simulink model "DCDC_4_5"  (R2012b)
settings: Solver=ode23  StartTime=0.0  StopTime=1370  FixedStep=0.1  MaxStep=0.005  RelTol=1e-6
undefined symbols (not defined in the file): Hydride, Metal, Nickel
libraries: powerlib x15, simulink x4, electricdrivelib x1
settings Model: Creator=Administrator  LastModifiedBy=Administrator
settings DataIOCC: SignalLoggingSaveFormat=ModelDataLogs
settings DebuggingCC: FcnCallInpInsideContextMsg=UseLocalSettings  StrictBusMsg=Warning
settings GRTTargetCC: CombineOutputUpdateFcns=off  GRTInterface=on

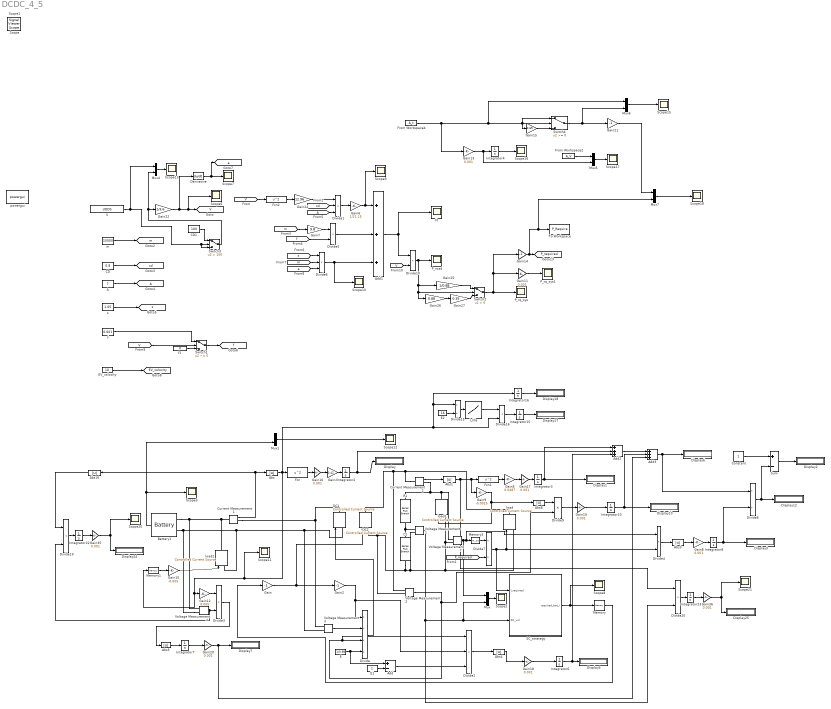
== system DCDC_4_5 ==
  A : Constant  Value=7
  Abs{,1,3..5,8,16} (7 alike) : Abs
  Add : Sum  Inputs=+-
  Add1 : Sum  Inputs=+++
  Add2 : Sum  Inputs=+++
  Add3 : Sum  Inputs=+++
  Battery1 : electricdrivelib/Extra Sources/Battery  BatType=Nickel-Metal-Hydride  ShowDetailedParameters=on  NomV=576  NomQ=160  SOC=90  PresetModel=off  MaxQ=17.2308  FullV=306.2712  Dis_rate=3.2  R=0.09  Normal_OP=15.3846  expZone="[282.0339           3.2]"  Dis_Char=off  current=[1.5 3]  Units=Ampere-hour  Batt_Tr=30
  C1 : powerlib/Elements/Series RLC Branch  LConnTagsString=__new0  RConnTagsString=__new0  BranchType=C  Resistance=1  Inductance=1e-3  SetiL0=off  InitialCurrent=0  Capacitance=14.1  Setx0=on  InitialVoltage=400  Measurements=Branch voltage
  CD : Constant  Value=0.8
  CD1 : Constant  Value=100
  Constant : Constant
  Current Measurement1 : powerlib/Measurements/Current Measurement  PhasorSimulation=off  OutputType=Complex  PSBequivalent=0
  Current Measurement2 : powerlib/Measurements/Current Measurement  PhasorSimulation=off  OutputType=Complex  PSBequivalent=0
  DC1 : powerlib/Electrical Sources/Controlled Current Source  Initialize=on  Source_Type=AC  Amplitude=0  Phase=0  Frequency=0  Measurements=None
  DC2 : powerlib/Electrical Sources/Controlled Current Source  Initialize=on  Source_Type=AC  Amplitude=0  Phase=0  Frequency=0  Measurements=None
  Derivative : Derivative
  Display{,1..4,6..7,10,12,17..18,24..25} (13 alike) : Display
  Divide : Product  Inputs=*/**
  Divide1 : Product  Inputs=***
  Divide{3..5,9..10,16,19..20} (8 alike) : Product  Inputs=**
  Divide15 : Product  Inputs=*/
  Divide2 : Product  Inputs=***
  Divide6 : Product  Inputs=***
  Divide7 : Product  Inputs=/*
  Divide8 : Product  Inputs=*/
  E : Constant  Value=1/0.98
  E1 : Constant
  E2 : Constant  Value=16
  EV_volocity : Constant  Value=10
  Fcn : Fcn  Expr=u^2
  Fcn1 : Fcn  Expr=u^2
  Fcn2 : Fcn  Expr=u^2
  From Workspace2 : FromWorkspace  VariableName=A_V  SampleTime=0
  From Workspace4 : FromWorkspace  VariableName=A_t  SampleTime=0
  Ft : Scope
      settings: SaveName=ScopeData9
  Gain{,2,14,21} (4 alike) : Gain  Gain=-1
  Gain10 : Gain  Gain=-0.005
  Gain{8,11,13,16..20,35..36} (10 alike) : Gain  Gain=0.001
  Gain12 : Gain  Gain=0.005
  Gain15 : Gain  Gain=0.65
  Gain22 : Gain  Gain=1/3.6
  Gain24 : Gain  Gain=12.96
  Gain25 : Gain  Gain=1/0.88
  Gain26 : Gain  Gain=0.88
  Gain27 : Gain  Gain=0.35
  Gain4 : Gain  Gain=0.42
  Gain5 : Gain  Gain=0.0487
  Gain6 : Gain  Gain=1/21.15
  Gain7 : Gain  Gain=9.8
  Gain9 : Gain  Gain=-0.0025
  I_life : Lookup  InputValues=[1,2,3,4,5]  Table=[1,1.0222,1.033,1.09,1.179]
  Integrator{2..4,6..8,10,15..16,22..23} (11 alike) : Integrator
  Memory : Memory
  Memory1 : Memory
  Memory3 : Memory  X0=380
  Mux{,1,4..7} (6 alike) : Mux  Inputs=2
  P_road : Scope
      settings: SaveName=P_road
  P_rq_sys : Scope
      settings: SaveName=ScopeData11
  P_rq_sys1 : Scope
      settings: SaveName=ScopeData10
  R1 : powerlib/Elements/Series RLC Branch  LConnTagsString=__new0  RConnTagsString=__new0  BranchType=R  Resistance=0.0487  Inductance=1e-3  SetiL0=off  InitialCurrent=0  Capacitance=1e-6  Setx0=off  InitialVoltage=0  Measurements=None
  SC_strategy : Subsystem
  Scope{2..3,6..13,15..18,20..21} (16 alike) : Scope
      Scope10 settings: SaveName=ScopeData12
      Scope11 settings: SaveName=ScopeData4
      Scope12 settings: TimeRange=206.5472513897466  YMin=-57.18262806236083  YMax=152.5055679287305
      Scope13 settings: SaveName=ScopeData8
      Scope15 settings: SaveName=ScopeData13
      Scope16 settings: SaveName=ScopeData14
      Scope17 settings: SaveName=ScopeData15
      Scope18 settings: SaveName=ScopeData16
      Scope2 settings: TimeRange=1600  YMin=240  YMax=420  SaveName=ScopeData2
      Scope20 settings: SaveName=ScopeData18
      Scope21 settings: SaveName=ScopeData19
      Scope3 settings: SaveName=ScopeData3
      Scope6 settings: SaveName=ScopeData17
      Scope7 settings: SaveName=ScopeData20
      Scope8 settings: SaveName=ScopeData5
      Scope9 settings: SaveName=ScopeData21
  Sum : Sum  Inputs=+-
  Switch1 : Switch  Criteria=u2 ~= 0
  Switch2 : Switch  Criteria=u2 > Threshold
  Switch3 : Switch  Criteria=u2 > Threshold  Threshold=100
  Switch4 : Switch
  To Workspace : ToWorkspace  VariableName=P_Require  SampleTime=-1
  V : FromWorkspace  VariableName=UDDS  SampleTime=0
  Voltage Measurement{1..4,7} (5 alike) : powerlib/Measurements/Voltage Measurement  PhasorSimulation=off  OutputType=Complex  PSBequivalent=0
  f : Constant  Value=0.001
  f1 : Constant  Value=0
  load : powerlib/Electrical Sources/Controlled Current Source  Initialize=on  Source_Type=AC  Amplitude=0  Phase=0  Frequency=0  Measurements=None
  load1 : powerlib/Electrical Sources/Controlled Current Source  Initialize=on  Source_Type=AC  Amplitude=0  Phase=0  Frequency=0  Measurements=None
  load2 : powerlib/Electrical Sources/Controlled Current Source  Initialize=on  Source_Type=AC  Amplitude=0  Phase=0  Frequency=0  Measurements=None
  m : Constant  Value=15000
  powergui : powerlib/powergui  Priority=1  SimulationMode=Discrete  SolverType=Tustin  SampleTime=0.01  frequency=60  SPID=off  DisableSnubberDevices=off  DisableRonSwitches=off  DisableVfSwitches=off  SwTol=0  Interpol=off  DisplayEquations=off  FunctionMessages=off  frequencyindice=0  Pbase=100e6  ErrMax=1e-4  Iterations=50  UnitsV=kV  UnitsW=MW  echomessages=off  HookPort=off  EnableUseOfTLC=off  x0status=blocks  RestoreLinks=warning  ResistiveCurrentMeasurement=off  Ylog=off  Xlog=on  ShowGrid=off  save=off  variable=ZData  ZoomFFT=off  StartTime=0.0  cycles=1  DisplayStyle=1  FreqAxis=off  MaxFrequency=1000  frequencyindicesteady=1  display=off  methode=off
  s : Constant  Value=1.05
  Scope : SignalViewerScope  IOType=viewer  RefreshTime=0.035000
  Scope1 : SignalViewerScope  IOType=viewer  RefreshTime=0.035000
  tag scope: A=global, EV_volocity=global, P_required=global, V=global, a=global, cd=global, f=global, m=global, s=global
  wires:
  Divide7/1 -> SC_strategy/1(I_requried), load/1, Divide4/2
  Battery1/1 -> Mux1/2, Scope3/1
  Voltage Measurement2/1 -> Divide/3, Divide2/1, Divide9/2
  Voltage Measurement1/1 -> Divide20/2, SC_strategy/2(SC_vol), Mux/2
  E/1 -> Divide/4, Add/1
  Voltage Measurement3/1 -> Divide/2
  Divide/1 -> DC1/1
  SC_strategy/1(required_bat_I) -> Memory/1, Scope8/1
  Memory/1 -> Gain/1
  Gain/1 -> DC2/1, Gain2/1
  Gain2/1 -> Divide/1, Divide2/2
  Current Measurement1/1 -> Abs/1, Abs16/1
  Current Measurement2/1 -> Abs1/1
  Abs/1 -> Fcn/1, Divide16/2, Divide15/1, Integrator16/1, Gain12/1, Memory1/1, Scope11/1
  Fcn/1 -> Gain16/1
  Gain4/1 -> Integrator2/1
  Integrator2/1 -> Display/1, Add2/2
  Fcn1/1 -> Gain5/1
  Gain5/1 -> Gain17/1
  Abs1/1 -> Fcn1/1, Gain9/1, Divide20/1
  Integrator3/1 -> Display1/1, Add2/1
  E1/1 -> Add/2
  Add/1 -> Divide2/3
  Abs4/1 -> Gain18/1
  Integrator6/1 -> Display4/1, Add2/3
  Divide2/1 -> Abs4/1
  Gain9/1 -> load1/1, Abs8/1
  Gain10/1 -> load2/1
  Voltage Measurement4/1 -> Divide3/2, Divide19/2
  Integrator7/1 -> Gain20/1
  Divide3/1 -> Abs5/1
  Abs5/1 -> Integrator7/1
  Gain12/1 -> Divide3/1
  [P_required] -> Divide7/2
  Voltage Measurement7/1 -> Divide4/1, Memory3/1, Mux/1
  Memory1/1 -> Gain10/1
  Memory3/1 -> Divide7/1
  Divide9/1 -> Gain19/1
  Integrator10/1 -> Display10/1, Add3/2
  Abs8/1 -> Divide9/1
  Divide4/1 -> Abs3/1
  Abs3/1 -> Gain8/1
  Integrator8/1 -> Display3/1, Divide8/2
  Gain8/1 -> Integrator8/1
  Gain16/1 -> Gain4/1
  Gain17/1 -> Integrator3/1
  Gain18/1 -> Integrator6/1
  Gain19/1 -> Integrator10/1
  Gain20/1 -> Display7/1, Add3/3
  Add2/1 -> Add3/1
  Add3/1 -> Divide8/1, Display6/1
  Divide8/1 -> Display12/1, Sum/2
  Mux1/1 -> Scope12/1
  Divide15/1 -> I_life/1
  E2/1 -> Divide15/2
  I_life/1 -> Divide16/1
  Divide16/1 -> Integrator15/1
  Integrator15/1 -> Display17/1
  Integrator16/1 -> Display18/1
  Divide19/1 -> Integrator22/1
  Integrator22/1 -> Gain35/1
  Gain35/1 -> Scope20/1, Display24/1
  Abs16/1 -> Divide19/1
  Divide20/1 -> Integrator23/1
  Integrator23/1 -> Gain36/1
  Gain36/1 -> Scope21/1, Display25/1
  Mux/1 -> Scope2/1
  V/1 -> Mux4/1, Switch3/3, Switch3/2
  m/1 -> [m]
  CD/1 -> [cd]
  A/1 -> [A]
  s/1 -> [s]
  Derivative/1 -> Scope7/1, [a]
  [V] -> Fcn2/1
  Fcn2/1 -> Gain24/1
  [cd] -> Divide1/2
  Divide1/1 -> Gain6/1
  Gain6/1 -> Add1/1, Scope9/1
  [m] -> Gain7/1
  Gain7/1 -> Divide5/1
  [f] -> Divide5/2
  [A] -> Divide1/3
  Divide5/1 -> Add1/2
  [s] -> Divide6/1
  [m] -> Divide6/2
  [a] -> Divide6/3
  Divide6/1 -> Add1/3, Scope10/1
  Add1/1 -> Ft/1, Divide10/1
  f/1 -> Switch1/1
  [V] -> Switch1/2
  f1/1 -> Switch1/3
  Switch1/1 -> [f]
  Gain22/1 -> Derivative/1, [V], Scope6/1
  [V] -> Divide10/2
  Gain24/1 -> Divide1/1
  Divide10/1 -> P_road/1, Gain25/1, Switch2/2, Gain26/1
  Gain25/1 -> Switch2/1
  Gain26/1 -> Gain27/1
  Switch2/1 -> P_rq_sys/1, Gain11/1, Gain14/1
  Gain27/1 -> Switch2/3
  EV_volocity/1 -> [EV_volocity]
  Gain14/1 -> Mux7/2, To Workspace/1, [P_required]
  Gain11/1 -> P_rq_sys1/1
  CD1/1 -> Switch3/1
  Switch3/1 -> Mux4/2, Gain22/1
  Mux4/1 -> Scope13/1
  Gain13/1 -> Integrator4/1, Mux5/2
  Integrator4/1 -> Scope16/1
  From Workspace4/1 -> Gain15/1, Switch4/1, Switch4/2, Mux6/1, Gain13/1
  From Workspace2/1 -> Mux5/1
  Mux5/1 -> Scope17/1
  Switch4/1 -> Gain21/1, Mux6/2
  Gain15/1 -> Switch4/3
  Mux6/1 -> Scope15/1
  Gain21/1 -> Mux7/1
  Mux7/1 -> Scope18/1
  Constant/1 -> Sum/1
  Sum/1 -> Display2/1
  connections:
  Current Measurement2/LConn1 -- load/RConn1 -- DC2/RConn1 -- Voltage Measurement2/LConn1
  C1/LConn1 -- Voltage Measurement1/LConn1 -- R1/RConn1
  load/LConn1 -- load1/LConn1 -- Voltage Measurement7/LConn2 -- DC2/LConn1 -- Voltage Measurement2/LConn2 -- C1/RConn1 -- Voltage Measurement1/LConn2
  Current Measurement1/RConn1 -- Voltage Measurement3/LConn1 -- DC1/RConn1
  Voltage Measurement4/LConn2 -- Battery1/LConn2 -- Voltage Measurement3/LConn2 -- DC1/LConn1 -- load2/LConn1
  Battery1/LConn1 -- Voltage Measurement4/LConn1 -- load2/RConn1 -- Current Measurement1/LConn1
  Voltage Measurement7/LConn1 -- load1/RConn1 -- Current Measurement2/RConn1 -- R1/LConn1

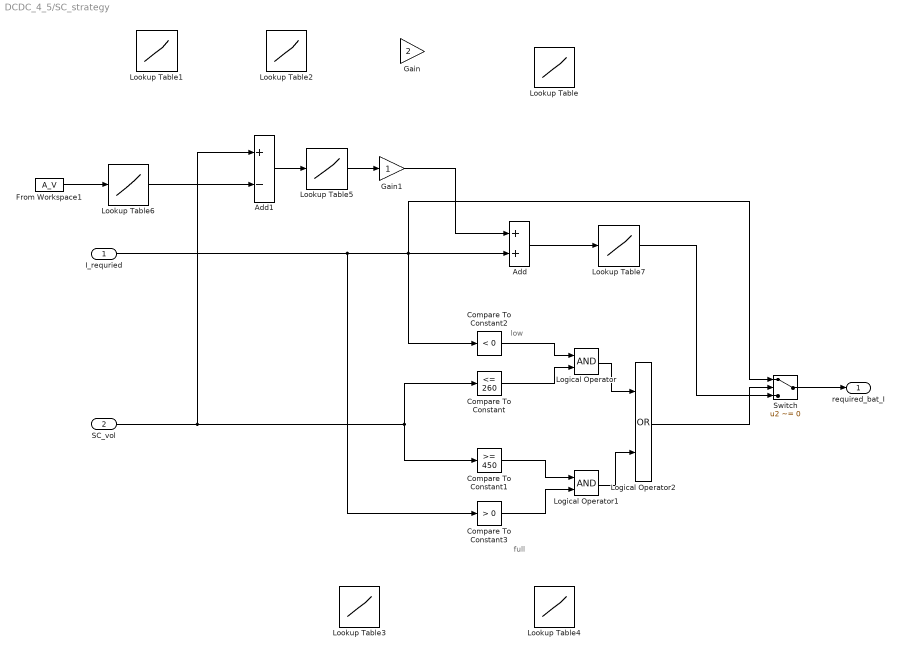
== system DCDC_4_5/SC_strategy ==
  note: full
  note: low
  I_requried : Inport
  SC_vol : Inport  Port=2
  Add : Sum
  Add1 : Sum  Inputs=+-
  Compare To Constant : simulink/Logic and Bit Operations/Compare To Constant  relop=<=  const=260  OutDataTypeStr=uint8  ZeroCross=off
  Compare To Constant1 : simulink/Logic and Bit Operations/Compare To Constant  relop=>=  const=450  OutDataTypeStr=uint8  ZeroCross=off
  Compare To Constant2 : simulink/Logic and Bit Operations/Compare To Constant  relop=<  const=0  OutDataTypeStr=uint8  ZeroCross=off
  Compare To Constant3 : simulink/Logic and Bit Operations/Compare To Constant  relop=>  const=0  OutDataTypeStr=uint8  ZeroCross=off
  From Workspace1 : FromWorkspace  VariableName=A_V  SampleTime=0
  Gain : Gain  Gain=2
  Gain1 : Gain
  Logical Operator : Logic  AllPortsSameDT=off  OutDataTypeStr=boolean
  Logical Operator1 : Logic  AllPortsSameDT=off  OutDataTypeStr=boolean
  Logical Operator2 : Logic  Operator=OR  AllPortsSameDT=off  OutDataTypeStr=boolean
  Lookup Table : Lookup  InputValues=[-260,-180,-100,-40,-20,-10,0,10,20,40,100,180,260]  Table=[-60,-30,-0,0,0,0,0,0,0,0,0,30,60]
  Lookup Table1 : Lookup  InputValues=[0,10,20,35,50,60]  Table=[390,380,370,355,335,260]
  Lookup Table2 : Lookup  InputValues=[-50,-30,-10,10,30,50]  Table=[-150,-50,-10,10,50,150]
  Lookup Table3 : Lookup  InputValues=[0,100,200,300,400,500,600,700,800,900,1000]  Table=|
      | [84.4	45.4072	44.31	42.7064	52.328	69.3768	140.104	182.304	172.176	163.736	151.92
      | ]
  Lookup Table4 : Lookup  InputValues=[0,100,200,300,400,500,600,700,800,900,1000]  Table=|
      | [10	5.38	5.25	5.06	6.2	8.22	16.6	21.6	20.4	19.4	18
      | ]
  Lookup Table5 : Lookup  InputValues=[-50,-30,-20,20,30,50]  Table=[-150,-50,0,0,50,150]
  Lookup Table6 : Lookup  InputValues=[0,10,20,35,50,60]  Table=[410,395,380,365,335,280]
  Lookup Table7 : Lookup  InputValues=[-300,-210,-150,-40,-20,-10,0,10,20,40,160,220,300]  Table=[-58,-57,-0,0,0,0,0,0,0,0,0,57,57]
  Switch : Switch  Criteria=u2 ~= 0
  required_bat_I : Outport
  wires:
  I_requried/1 -> Switch/1, Add/2, Compare To Constant2/1, Compare To Constant3/1
  Lookup Table7/1 -> Switch/3
  SC_vol/1 -> Add1/1, Compare To Constant/1, Compare To Constant1/1
  Compare To Constant/1 -> Logical Operator/2
  Compare To Constant2/1 -> Logical Operator/1
  Compare To Constant1/1 -> Logical Operator1/1
  Compare To Constant3/1 -> Logical Operator1/2
  Logical Operator/1 -> Logical Operator2/1
  Logical Operator1/1 -> Logical Operator2/2
  Logical Operator2/1 -> Switch/2
  Switch/1 -> required_bat_I/1
  Add/1 -> Lookup Table7/1
  Add1/1 -> Lookup Table5/1
  Lookup Table6/1 -> Add1/2
  Gain1/1 -> Add/1
  From Workspace1/1 -> Lookup Table6/1
  Lookup Table5/1 -> Gain1/1
